simulink model "example_model"  (R2021a)
settings: Solver=FixedStepDiscrete  StartTime=0.0  StopTime=10  RelTol=1e-3
undefined symbols (not defined in the file): f
libraries: instrumentlib x6
settings Model: EnablePacing=on  Creator=huid  LastModifiedBy=huid

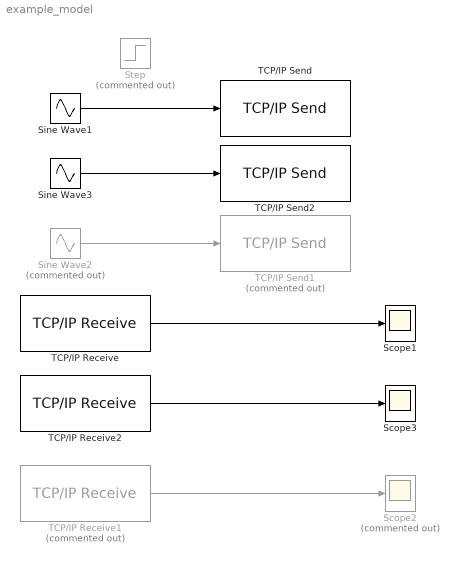
== system example_model ==
  Scope1 : Scope
  Scope2 : Scope  Commented=on
  Scope3 : Scope
  Sine Wave1 : Sin  Amplitude=2  Frequency=2*pi/10  SampleTime=0.05
  Sine Wave2 : Sin  Commented=on  Amplitude=2  Frequency=2*pi/10  SampleTime=0.05
  Sine Wave3 : Sin  Amplitude=2  Frequency=2*pi/10  SampleTime=0.05
  Step : Step  Commented=on  SampleTime=0.1
  TCP/IP Receive : instrumentlib/TCP//IP Receive  Priority=2  Host=59.78.14.250  Port=50000  DataSize="[1  1]"  EnableBlockingMode=on  Timeout=10  SampleTime=0.1  DataType=double  ByteOrder=BigEndian  ASCIIFormatting=%f,  Terminator=LF
  TCP/IP Receive1 : instrumentlib/TCP//IP Receive  Priority=2  Commented=on  Host=59.78.6.82  Port=50000  DataSize="[1  1]"  EnableBlockingMode=on  Timeout=60  SampleTime=0.1  DataType=double  ByteOrder=BigEndian  ASCIIFormatting=%f,  Terminator=LF
  TCP/IP Receive2 : instrumentlib/TCP//IP Receive  Priority=2  Host=59.78.4.161  Port=50001  DataSize="[1  1]"  EnableBlockingMode=on  Timeout=60  SampleTime=0.1  DataType=double  ByteOrder=BigEndian  ASCIIFormatting=%f,  Terminator=LF
  TCP/IP Send : instrumentlib/TCP//IP Send  Priority=1  Host=59.78.14.250  Port=50000  EnableBlockingMode=on  Timeout=10  ByteOrder=BigEndian  TransferDelay=on
  TCP/IP Send1 : instrumentlib/TCP//IP Send  Priority=1  Commented=on  Host=59.78.6.82  Port=50000  EnableBlockingMode=on  Timeout=10  ByteOrder=BigEndian  TransferDelay=on
  TCP/IP Send2 : instrumentlib/TCP//IP Send  Priority=1  Host=59.78.4.161  Port=50001  EnableBlockingMode=on  Timeout=10  ByteOrder=BigEndian  TransferDelay=on
  wires:
  Sine Wave1/1 -> TCP/IP Send/1
  TCP/IP Receive/1 -> Scope1/1
  TCP/IP Receive1/1 -> Scope2/1
  TCP/IP Receive2/1 -> Scope3/1
  Sine Wave2/1 -> TCP/IP Send1/1
  Sine Wave3/1 -> TCP/IP Send2/1
